simulink model "iiwaStiffnessLearning"  (R2015b)
settings: Solver=VariableStepAuto  StartTime=0.0  StopTime=inf  FixedStep=0.01  RelTol=1e-3
values from neighbouring files (symbols this model uses):
  dt = 0.15    [genKUKATrajectory.m]
  T = 10    [genKUKATrajectory.m]
undefined symbols (not defined in the file or in its folder): constMean, dt_pilco, indices, initRollout, jj, multTargets, plant, policy, Pose, seedMatrix, Stiffness, varTargets
libraries: robotlib x10, realtime_pacer_lib x2
settings Model: Creator=victor  LastModifiedBy=localadmin
settings SolverCC: ZeroCrossAlgorithm=Adaptive  AutoInsertRateTranBlk=on
settings OptimizationCC: OptimizeModelRefInitCode=on  LifeSpan=Inf  MaxStackSize=64
settings HardwareCC: ProdBitPerLong=64  ProdHWDeviceType=Intel->x86-64 (Linux 64)
settings RTWCC: SystemTargetFile=ert.tlc  TemplateMakefile=ert_default_tmf  Description=Embedded Coder  Toolchain=Catkin  TargetLang=C++
settings ERTTargetCC: GenerateSampleERTMain=on  MultiInstanceERTCode=on  CodeInterfacePackaging=C++ class  RootIOFormat=Structure reference

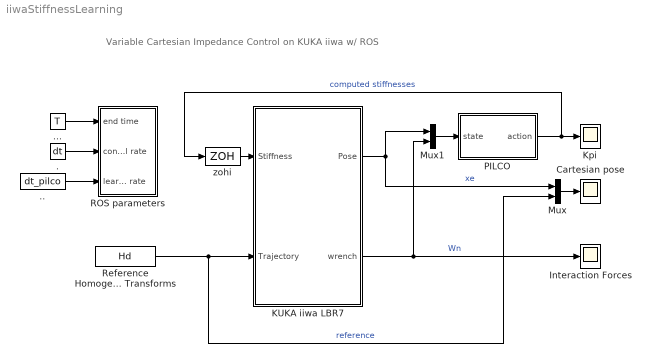
== system iiwaStiffnessLearning ==
  note: Variable Cartesian Impedance Control on KUKA iiwa w/ ROS
  . : Constant  Value=dt
  .. : Constant  Value=dt_pilco
  ... : Constant  Value=T
  Cartesian pose : Scope
  Interaction Forces : Scope
  KUKA iiwa LBR7 : Subsystem
  Kpi : Scope
  Mux : Mux  Inputs=2
  Mux1 : Mux  Inputs=2
  PILCO : Subsystem
  ROS parameters : Subsystem
  Reference Homogenous Transforms : FromWorkspace  VariableName=Hd  SampleTime=dt  OutputAfterFinalValue=Holding final value
  zohi : ZeroOrderHold  SampleTime=dt
  wires:
  zohi/1 -> KUKA iiwa LBR7/1(Stiffness)
  KUKA iiwa LBR7/1(Pose) -> Mux1/1, Mux/1  "xe"
  Mux1/1 -> PILCO/1(state)
  PILCO/1(action) -> zohi/1, Kpi/1  "computed stiffnesses"
  Reference Homogenous Transforms/1 -> KUKA iiwa LBR7/2(Trajectory), Mux/2  "reference"
  Mux/1 -> Cartesian pose/1
  KUKA iiwa LBR7/2(wrench) -> Mux1/2, Interaction Forces/1  "Wn"
  .../1 -> ROS parameters/1(end time)
  ./1 -> ROS parameters/2(control rate)
  ../1 -> ROS parameters/3(learning rate)

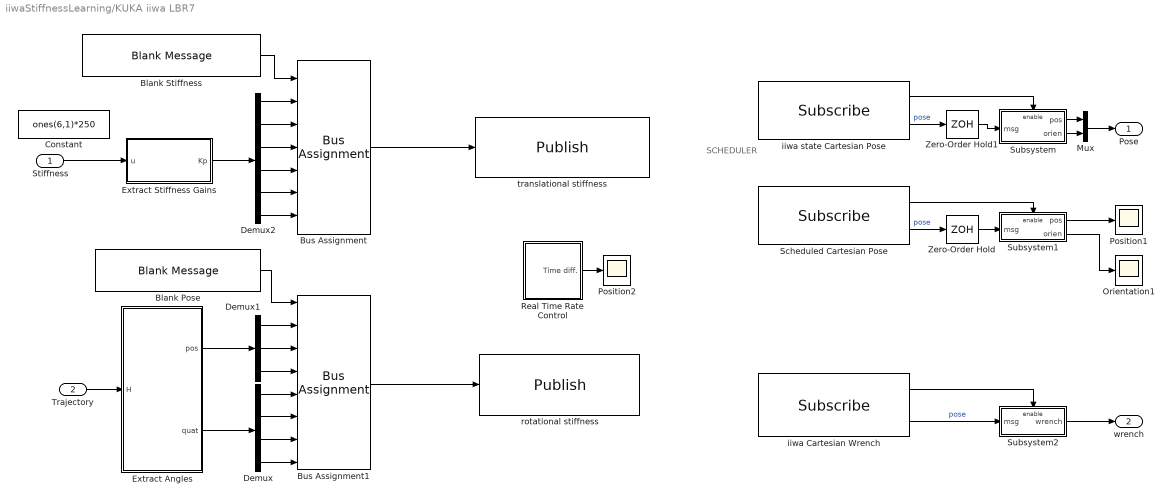
== system iiwaStiffnessLearning/KUKA iiwa LBR7 ==
  note: SCHEDULER
  Stiffness : Inport
  Trajectory : Inport  Port=2
  Blank Pose : robotlib/Blank Message  SourceLibraryInfo=This block requires Robotics System Toolbox  messageType=geometry_msgs/PoseStamped  SampleTime=inf
  Blank Stiffness : robotlib/Blank Message  SourceLibraryInfo=This block requires Robotics System Toolbox  messageType=iiwa_msgs/CartesianStiffness  SampleTime=inf
  Bus Assignment : BusAssignment  AssignedSignals=Stiffness.X,Stiffness.Y,Stiffness.Z,Stiffness.A,Stiffness.B,Stiffness.C
  Bus Assignment1 : BusAssignment  AssignedSignals=Pose.Position.X,Pose.Position.Y,Pose.Position.Z,Pose.Orientation.X,Pose.Orientation.Y,Pose.Orientation.Z,Pose.Orientation.W
  Constant : Constant  Value=ones(6,1)*250
  Demux : Demux
  Demux1 : Demux  Outputs=3
  Demux2 : Demux  Outputs=6
  Extract Angles : MATLAB Function  TreatAsAtomicUnit=on
  Extract Stiffness Gains : MATLAB Function  TreatAsAtomicUnit=on
  Mux : Mux  Inputs=2
  Orientation1 : Scope
  Position1 : Scope
  Position2 : Scope
  Real Time Rate Control : Subsystem
  Scheduled Cartesian Pose : robotlib/Subscribe  SourceLibraryInfo=This block requires Robotics System Toolbox  topicSource=Specify your own  topic=/scheduler/state/CartesianPose  messageType=geometry_msgs/PoseStamped  sampleTime=-1  messageQueueLength=1
  Subsystem : Subsystem
  Subsystem1 : Subsystem
  Subsystem2 : Subsystem
  Zero-Order Hold : ZeroOrderHold  SampleTime=0.1
  Zero-Order Hold1 : ZeroOrderHold  SampleTime=0.01
  iiwa Cartesian Wrench : robotlib/Subscribe  SourceLibraryInfo=This block requires Robotics System Toolbox  topicSource=Specify your own  topic=/iiwa/state/CartesianWrench  messageType=geometry_msgs/WrenchStamped  sampleTime=-1  messageQueueLength=1
  iiwa state Cartesian Pose : robotlib/Subscribe  SourceLibraryInfo=This block requires Robotics System Toolbox  topicSource=Specify your own  topic=/iiwa/state/CartesianPose  messageType=geometry_msgs/PoseStamped  sampleTime=-1  messageQueueLength=1
  rotational stiffness : robotlib/Publish  SourceLibraryInfo=This block requires Robotics System Toolbox  topicSource=Specify your own  topic=/matlab/actions/CartesianPose  messageType=geometry_msgs/Vector3Stamped  messageQueueLength=1
  translational stiffness : robotlib/Publish  SourceLibraryInfo=This block requires Robotics System Toolbox  topicSource=Specify your own  topic=/matlab/actions/CartesianStiffness  messageType=geometry_msgs/Vector3Stamped  messageQueueLength=1
  Pose : Outport
  wrench : Outport  Port=2
  wires:
  Blank Stiffness/1 -> Bus Assignment/1
  Bus Assignment/1 -> translational stiffness/1
  Bus Assignment1/1 -> rotational stiffness/1
  iiwa state Cartesian Pose/2 -> Zero-Order Hold1/1  "pose"
  iiwa state Cartesian Pose/1 -> Subsystem/Enable
  Scheduled Cartesian Pose/2 -> Zero-Order Hold/1  "pose"
  Subsystem1/1(pos) -> Position1/1
  Subsystem1/2(orien) -> Orientation1/1
  Scheduled Cartesian Pose/1 -> Subsystem1/Enable
  Zero-Order Hold/1 -> Subsystem1/1(msg)
  Zero-Order Hold1/1 -> Subsystem/1(msg)
  Blank Pose/1 -> Bus Assignment1/1
  Demux/1 -> Bus Assignment1/5
  Demux/2 -> Bus Assignment1/6
  Demux/3 -> Bus Assignment1/7
  Demux/4 -> Bus Assignment1/8
  Demux1/1 -> Bus Assignment1/2
  Demux1/2 -> Bus Assignment1/3
  Demux1/3 -> Bus Assignment1/4
  Trajectory/1 -> Extract Angles/1(H)
  Demux2/4 -> Bus Assignment/5
  Demux2/6 -> Bus Assignment/7
  Demux2/5 -> Bus Assignment/6
  Demux2/3 -> Bus Assignment/4
  Demux2/2 -> Bus Assignment/3
  Demux2/1 -> Bus Assignment/2
  Stiffness/1 -> Extract Stiffness Gains/1(u)
  Mux/1 -> Pose/1
  Subsystem/1(pos) -> Mux/1
  Subsystem/2(orien) -> Mux/2
  iiwa Cartesian Wrench/2 -> Subsystem2/1(msg)  "pose"
  iiwa Cartesian Wrench/1 -> Subsystem2/Enable
  Subsystem2/1(wrench) -> wrench/1
  Extract Stiffness Gains/1(Kp) -> Demux2/1
  Extract Angles/1(pos) -> Demux1/1
  Extract Angles/2(quat) -> Demux/1
  Real Time Rate Control/1(Time diff.) -> Position2/1

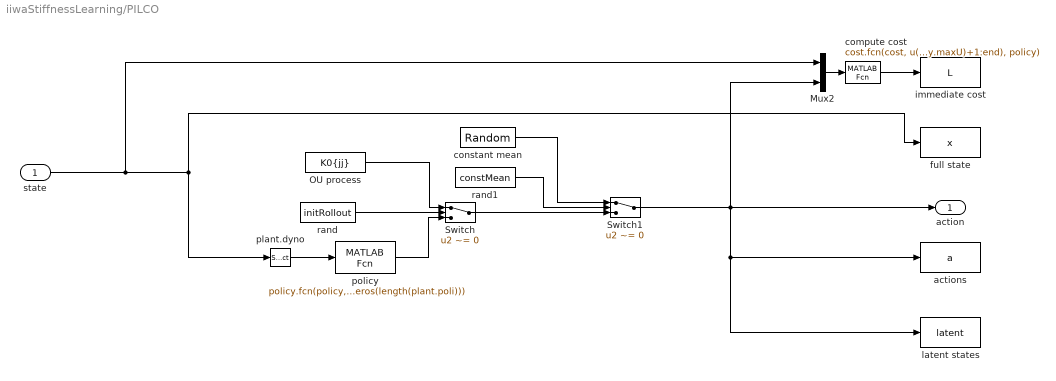
== system iiwaStiffnessLearning/PILCO ==
  state : Inport
  Mux2 : Mux  Inputs=2
  OU process : FromWorkspace  VariableName=K0{jj}  SampleTime=dt_pilco
  Switch : Switch  Criteria=u2 ~= 0
  Switch1 : Switch  Criteria=u2 ~= 0
  actions : ToWorkspace  VariableName=a  SampleTime=dt_pilco
  compute cost : MATLABFcn  MATLABFcn=cost.fcn(cost, u(plant.dyno), zeros(length(plant.dyno)), u(end-length(policy.maxU)+1:end), policy)  OutputDimensions=1  Output1D=off
  constant mean : RandomNumber  Mean=multTargets(jj,:)  Variance=varTargets  Seed=seedMatrix(jj,:)  SampleTime=dt_pilco
  full state : ToWorkspace  VariableName=x  SampleTime=dt_pilco
  immediate cost : ToWorkspace  VariableName=L  SampleTime=dt_pilco
  latent states : ToWorkspace  VariableName=latent  SampleTime=dt_pilco
  plant.dyno : Selector  InputPortWidth=length(indices)  IndexOptions=Index vector (dialog)  Indices=plant.dyno  OutputSizes=1
  policy : MATLABFcn  MATLABFcn=policy.fcn(policy, u(plant.poli), zeros(length(plant.poli)))
  rand : Constant  Value=initRollout
  rand1 : Constant  Value=constMean
  action : Outport
  wires:
  Switch1/1 -> latent states/1, actions/1, action/1, Mux2/2
  compute cost/1 -> immediate cost/1
  plant.dyno/1 -> policy/1
  rand/1 -> Switch/2
  policy/1 -> Switch/3
  OU process/1 -> Switch/1
  Mux2/1 -> compute cost/1
  state/1 -> Mux2/1, full state/1, plant.dyno/1
  rand1/1 -> Switch1/2
  constant mean/1 -> Switch1/1
  Switch/1 -> Switch1/3

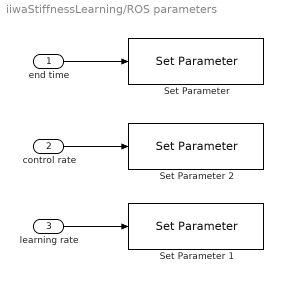
== system iiwaStiffnessLearning/ROS parameters ==
  end time : Inport
  control rate : Inport  Port=2
  learning rate : Inport  Port=3
  Set Parameter : robotlib/Set Parameter  SourceLibraryInfo=This block requires Robotics System Toolbox  ParameterSource=Specify your own  ParameterName=/terminalTime  ParameterType=double  ModelName=iiwaStiffnessLearning  BlockId=ParamSet_iiwaStiffnessLearning_216
  Set Parameter 1 : robotlib/Set Parameter  SourceLibraryInfo=This block requires Robotics System Toolbox  ParameterSource=Specify your own  ParameterName=/learningRate  ParameterType=double  ModelName=iiwaStiffnessLearning  BlockId=ParamSet_iiwaStiffnessLearning_223
  Set Parameter 2 : robotlib/Set Parameter  SourceLibraryInfo=This block requires Robotics System Toolbox  ParameterSource=Specify your own  ParameterName=/controlRate  ParameterType=double  ModelName=iiwaStiffnessLearning  BlockId=ParamSet_iiwaStiffnessLearning_221
  wires:
  end time/1 -> Set Parameter/1
  control rate/1 -> Set Parameter 2/1
  learning rate/1 -> Set Parameter 1/1

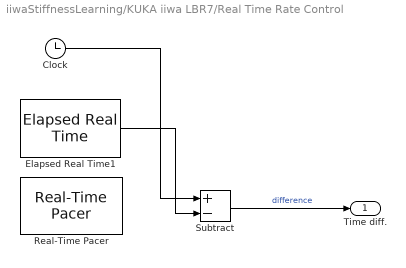
== system iiwaStiffnessLearning/KUKA iiwa LBR7/Real Time Rate Control ==
  Clock : Clock
  Elapsed Real Time1 : realtime_pacer_lib/Elapsed Real Time
  Real-Time Pacer : realtime_pacer_lib/Real-Time Pacer  simTimePerRealTime=1
  Subtract : Sum  Inputs=+-
  Time diff. : Outport
  wires:
  Elapsed Real Time1/1 -> Subtract/2
  Subtract/1 -> Time diff./1  "difference"
  Clock/1 -> Subtract/1

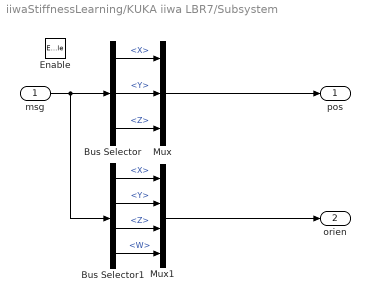
== system iiwaStiffnessLearning/KUKA iiwa LBR7/Subsystem ==
  msg : Inport
  Enable : EnablePort
  Bus Selector : BusSelector  OutputSignals=Pose.Position.X,Pose.Position.Y,Pose.Position.Z
  Bus Selector1 : BusSelector  OutputSignals=Pose.Orientation.X,Pose.Orientation.Y,Pose.Orientation.Z,Pose.Orientation.W
  Mux : Mux  Inputs=3
  Mux1 : Mux
  pos : Outport
  orien : Outport  Port=2
  wires:
  Bus Selector1/2 -> Mux1/2  "<Y>"
  Bus Selector1/4 -> Mux1/4  "<W>"
  Bus Selector/3 -> Mux/3  "<Z>"
  Bus Selector/1 -> Mux/1  "<X>"
  Bus Selector/2 -> Mux/2  "<Y>"
  Bus Selector1/3 -> Mux1/3  "<Z>"
  Mux1/1 -> orien/1
  Bus Selector1/1 -> Mux1/1  "<X>"
  Mux/1 -> pos/1
  msg/1 -> Bus Selector1/1, Bus Selector/1

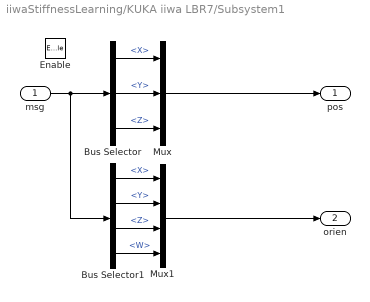
== system iiwaStiffnessLearning/KUKA iiwa LBR7/Subsystem1 ==
  msg : Inport
  Enable : EnablePort
  Bus Selector : BusSelector  OutputSignals=Pose.Position.X,Pose.Position.Y,Pose.Position.Z
  Bus Selector1 : BusSelector  OutputSignals=Pose.Orientation.X,Pose.Orientation.Y,Pose.Orientation.Z,Pose.Orientation.W
  Mux : Mux  Inputs=3
  Mux1 : Mux
  pos : Outport
  orien : Outport  Port=2
  wires:
  Bus Selector1/2 -> Mux1/2  "<Y>"
  Bus Selector1/4 -> Mux1/4  "<W>"
  Bus Selector/3 -> Mux/3  "<Z>"
  Bus Selector/1 -> Mux/1  "<X>"
  Bus Selector/2 -> Mux/2  "<Y>"
  Bus Selector1/3 -> Mux1/3  "<Z>"
  Mux1/1 -> orien/1
  Bus Selector1/1 -> Mux1/1  "<X>"
  Mux/1 -> pos/1
  msg/1 -> Bus Selector1/1, Bus Selector/1

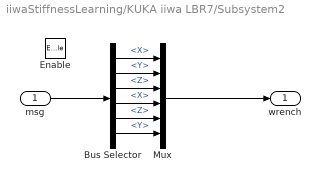
== system iiwaStiffnessLearning/KUKA iiwa LBR7/Subsystem2 ==
  msg : Inport
  Enable : EnablePort
  Bus Selector : BusSelector  OutputSignals=Wrench.Force.X,Wrench.Force.Y,Wrench.Force.Z,Wrench.Torque.X,Wrench.Torque.Z,Wrench.Torque.Y
  Mux : Mux  Inputs=6
  wrench : Outport
  wires:
  Bus Selector/3 -> Mux/3  "<Z>"
  Bus Selector/1 -> Mux/1  "<X>"
  Bus Selector/2 -> Mux/2  "<Y>"
  Mux/1 -> wrench/1
  msg/1 -> Bus Selector/1
  Bus Selector/4 -> Mux/4  "<X>"
  Bus Selector/5 -> Mux/5  "<Z>"
  Bus Selector/6 -> Mux/6  "<Y>"

== matlab function iiwaStiffnessLearning/KUKA iiwa LBR7/Extract Angles ==
  data: H input size=[3 1]; pos output size=[6 1]; quat output
function [pos, quat] = minimRep(H)
%# convert transformation matrix into quaternion

pos = transl(H);

quat = tform2quat(H);

== matlab function iiwaStiffnessLearning/KUKA iiwa LBR7/Extract Stiffness Gains ==
  data: u input size=[3 1]; Kp output size=[6 1]
function Kp = arrangeGains(u)
%# arranges gains stiffness gains in suitable manner. 
% !! HARD CODED !! change for different scenarios !@!@

Kp = [u(1), u(2), u(2), u(3), u(3), u(3)]';
